simulink model "task1"  (R2022b)
settings: Solver=FixedStepAuto  StartTime=0.0  StopTime=7  RelTol=1e-8
undefined symbols (not defined in the file): a0, a1, a2, b0, b1, b2
settings Model: Creator=anton  LastModifiedBy=anton
settings DataIOCC: ExternalInput=data  LoadExternalInput=on

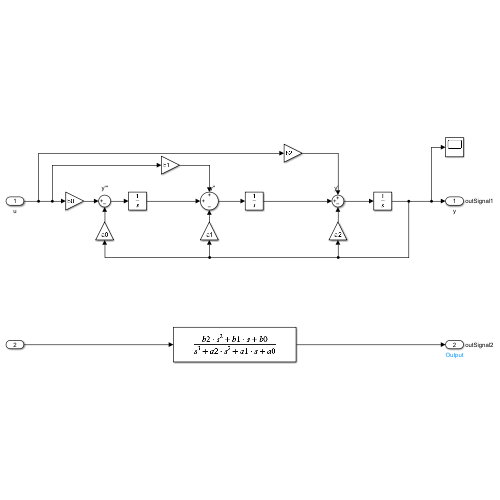
[thumbnail: Simulink's stored preview of the top-level diagram]
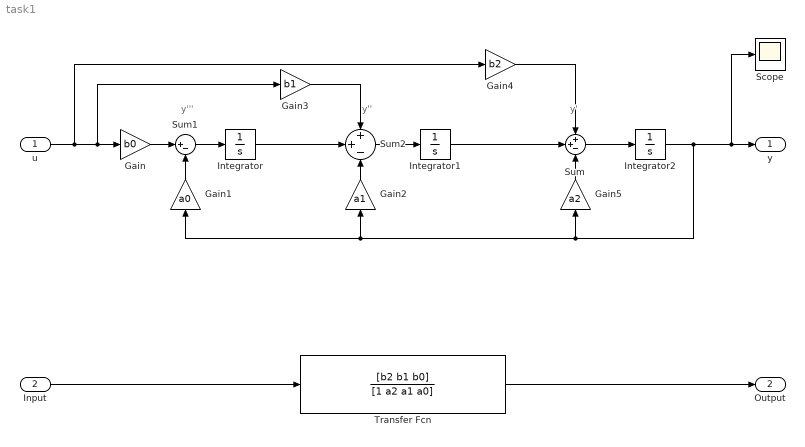
== system task1 ==
  note: y'''
  note: y''
  note: y'
  u : Inport
  Input : Inport  Port=2  PortDimensions=1
  Gain : Gain  Gain=b0
  Gain1 : Gain  Gain=a0
  Gain2 : Gain  Gain=a1
  Gain3 : Gain  Gain=b1
  Gain4 : Gain  Gain=b2
  Gain5 : Gain  Gain=a2
  Integrator : Integrator
  Integrator1 : Integrator
  Integrator2 : Integrator
  Scope : Scope
  Sum : Sum  Inputs=++-
  Sum1 : Sum  Inputs=|+-
  Sum2 : Sum  Inputs=++-
  Transfer Fcn : TransferFcn  Numerator=[b2 b1 b0]  Denominator=[1 a2 a1 a0]
  y : Outport  SignalName=outSignal1
  Output : Outport  Port=2  SignalName=outSignal2
  wires:
  Integrator2/1 -> Gain2/1, Gain1/1, Gain5/1, Scope/1, y/1
  Sum1/1 -> Integrator/1
  Gain/1 -> Sum1/1
  u/1 -> Gain4/1, Gain3/1, Gain/1
  Gain1/1 -> Sum1/2
  Sum2/1 -> Integrator1/1
  Gain3/1 -> Sum2/1
  Sum/1 -> Integrator2/1
  Gain4/1 -> Sum/1
  Input/1 -> Transfer Fcn/1
  Transfer Fcn/1 -> Output/1
  Gain2/1 -> Sum2/3
  Integrator/1 -> Sum2/2
  Gain5/1 -> Sum/3
  Integrator1/1 -> Sum/2
